simulink model "sim_sistema_2_observador"  (Simulink 7.5)
settings: Solver=ode3  StartTime=0.0  StopTime=15  FixedStep=1e-4  RelTol=1e-3
values from neighbouring files (symbols this model uses):
  B = sis.b    [sistema_2_observador.m]
  C = sis.c    [sistema_2_observador.m]
  K = acker(sis.a,sis.b,J)    [sistema_2.m]    (also in sistema_2_observador.m)
  Ke = phi*inv(obs)*col    [sistema_2_observador.m]
  sis = ss(sis)    [sistema_2.m]    (also in sistema_2_observador.m)
settings Model: Creator=taniel.franklin  LastModifiedBy=taniel.franklin

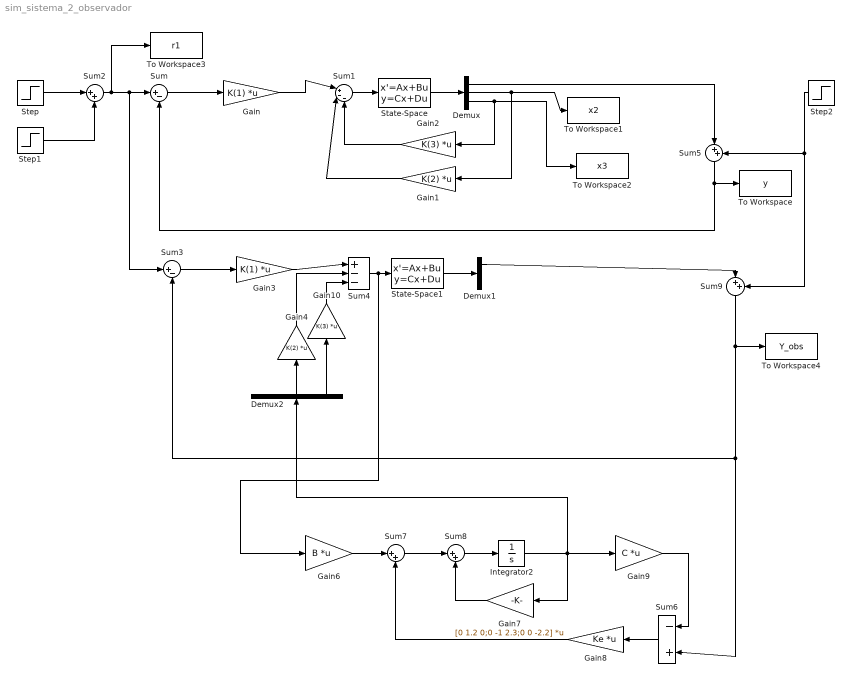
== system sim_sistema_2_observador ==
  Demux : Demux  Outputs=3
  Demux1 : Demux  Outputs=3
  Demux2 : Demux  Outputs=3
  Gain : Gain  Gain=K(1)  Multiplication=Matrix(K*u)  ParameterDataType=fixdt(1, 16)  ParameterScaling=2^0  OutDataType=fixdt(1, 16)  OutScaling=2^0
  Gain1 : Gain  Gain=K(2)  Multiplication=Matrix(K*u)  ParameterDataType=fixdt(1, 16)  ParameterScaling=2^0  OutDataType=fixdt(1, 16)  OutScaling=2^0
  Gain10 : Gain  Gain=K(3)  Multiplication=Matrix(K*u)  ParameterDataType=fixdt(1, 16)  ParameterScaling=2^0  OutDataType=fixdt(1, 16)  OutScaling=2^0
  Gain2 : Gain  Gain=K(3)  Multiplication=Matrix(K*u)  ParameterDataType=fixdt(1, 16)  ParameterScaling=2^0  OutDataType=fixdt(1, 16)  OutScaling=2^0
  Gain3 : Gain  Gain=K(1)  Multiplication=Matrix(K*u)  ParameterDataType=fixdt(1, 16)  ParameterScaling=2^0  OutDataType=fixdt(1, 16)  OutScaling=2^0
  Gain4 : Gain  Gain=K(2)  Multiplication=Matrix(K*u)  ParameterDataType=fixdt(1, 16)  ParameterScaling=2^0  OutDataType=fixdt(1, 16)  OutScaling=2^0
  Gain6 : Gain  Gain=B  Multiplication=Matrix(K*u)  ParameterDataType=fixdt(1, 16)  ParameterScaling=2^0  OutDataType=fixdt(1, 16)  OutScaling=2^0
  Gain7 : Gain  Gain=[0 1.2 0;0 -1 2.3;0 0 -2.2]  Multiplication=Matrix(K*u)  ParameterDataType=fixdt(1, 16)  ParameterScaling=2^0  OutDataType=fixdt(1, 16)  OutScaling=2^0
  Gain8 : Gain  Gain=Ke  Multiplication=Matrix(K*u)  ParameterDataType=fixdt(1, 16)  ParameterScaling=2^0  OutDataType=fixdt(1, 16)  OutScaling=2^0
  Gain9 : Gain  Gain=C  Multiplication=Matrix(K*u)  ParameterDataType=fixdt(1, 16)  ParameterScaling=2^0  OutDataType=fixdt(1, 16)  OutScaling=2^0
  Integrator2 : Integrator
  State-Space : StateSpace  A=sis.A  B=sis.B  C=eye(3)  D=[0;0;0]
  State-Space1 : StateSpace  A=sis.A  B=sis.B  C=eye(3)  D=[0;0;0]
  Step : Step  Time=0.2  SampleTime=0
  Step1 : Step  Time=5  SampleTime=0
  Step2 : Step  Time=9  After=0.5  SampleTime=0
  Sum : Sum  Inputs=|+-  OutDataType=fixdt(1, 16)  OutScaling=2^0
  Sum1 : Sum  Inputs=|+--  OutDataType=fixdt(1, 16)  OutScaling=2^0
  Sum{2,5,7..9} (5 alike) : Sum  Inputs=|++  OutDataType=fixdt(1, 16)  OutScaling=2^0
  Sum3 : Sum  Inputs=|+-  OutDataType=fixdt(1, 16)  OutScaling=2^0
  Sum4 : Sum  Inputs=|+--  OutDataType=fixdt(1, 16)  OutScaling=2^0
  Sum6 : Sum  Inputs=|-+  OutDataType=fixdt(1, 16)  OutScaling=2^0
  To Workspace : ToWorkspace  VariableName=y  SampleTime=-1  SaveFormat=Structure With Time
  To Workspace1 : ToWorkspace  VariableName=x2  SampleTime=-1  SaveFormat=Structure With Time
  To Workspace2 : ToWorkspace  VariableName=x3  SampleTime=-1  SaveFormat=Structure With Time
  To Workspace3 : ToWorkspace  VariableName=r1  SampleTime=-1  SaveFormat=Structure With Time
  To Workspace4 : ToWorkspace  VariableName=Y_obs  SampleTime=-1  SaveFormat=Structure With Time
  wires:
  State-Space/1 -> Demux/1
  Demux/2 -> To Workspace1/1, Gain1/1
  Demux/3 -> To Workspace2/1, Gain2/1
  Gain/1 -> Sum1/1
  Sum/1 -> Gain/1
  Sum1/1 -> State-Space/1
  Gain1/1 -> Sum1/2
  Gain2/1 -> Sum1/3
  Step/1 -> Sum2/1
  Step1/1 -> Sum2/2
  Sum2/1 -> To Workspace3/1, Sum/1, Sum3/1
  Demux/1 -> Sum5/1
  State-Space1/1 -> Demux1/1
  Gain3/1 -> Sum4/1
  Sum3/1 -> Gain3/1
  Sum4/1 -> State-Space1/1, Gain6/1
  Sum6/1 -> Gain8/1
  Gain8/1 -> Sum7/2
  Gain6/1 -> Sum7/1
  Sum8/1 -> Integrator2/1
  Sum7/1 -> Sum8/1
  Integrator2/1 -> Gain7/1, Gain9/1, Demux2/1
  Gain7/1 -> Sum8/2
  Gain9/1 -> Sum6/1
  Demux2/3 -> Gain10/1
  Demux2/2 -> Gain4/1
  Gain10/1 -> Sum4/3
  Gain4/1 -> Sum4/2
  Sum5/1 -> Sum/2, To Workspace/1
  Step2/1 -> Sum5/2, Sum9/2
  Demux1/1 -> Sum9/1
  Sum9/1 -> To Workspace4/1, Sum3/2, Sum6/2
